simulink model "SchematT"  (R2018b)
settings: Solver=VariableStepAuto  StartTime=0.0  StopTime=10.0  RelTol=1e-3
libraries: simulink_extras x2
settings Model: Creator=bartl  LastModifiedBy=bartl

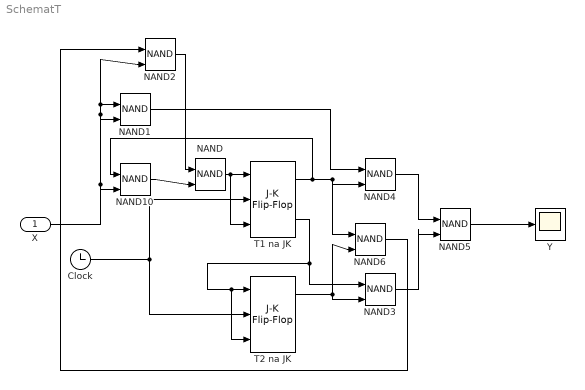
== system SchematT ==
  X : Inport
  Clock : Clock
  NAND{,1..6,10} (8 alike) : Logic  Operator=NAND  IconShape=distinctive  AllPortsSameDT=off  OutDataTypeStr=boolean
  T1 na JK : simulink_extras/Flip Flops/J-K Flip-Flop  initial_condition=0
      settings: SourceProductName=Simulink
  T2 na JK : simulink_extras/Flip Flops/J-K Flip-Flop  initial_condition=0
      settings: SourceProductName=Simulink
  Y : Scope
  wires:
  T1 na JK/2 -> NAND3/1, T2 na JK/3, T2 na JK/1
  Clock/1 -> T2 na JK/2, T1 na JK/2
  NAND/1 -> T1 na JK/3, T1 na JK/1
  T2 na JK/1 -> NAND6/2, NAND3/2
  T1 na JK/1 -> NAND10/1, NAND4/2, NAND6/1
  X/1 -> NAND10/2, NAND1/1, NAND2/2, NAND1/2
  NAND1/1 -> NAND4/1
  NAND4/1 -> NAND5/1
  NAND3/1 -> NAND5/2
  NAND5/1 -> Y/1
  NAND10/1 -> NAND/2
  NAND6/1 -> NAND2/1
  NAND2/1 -> NAND/1
